simulink model "the_museum"  (R2016b)
settings: Solver=VariableStepAuto  StartTime=0.0  StopTime=10.0  RelTol=1e-3
undefined symbols (not defined in the file or in its folder): Lb, Lf, Lu, RobotStruct
libraries: simulink x1
settings Model: Creator=niekbeckers  LastModifiedBy=Labuser

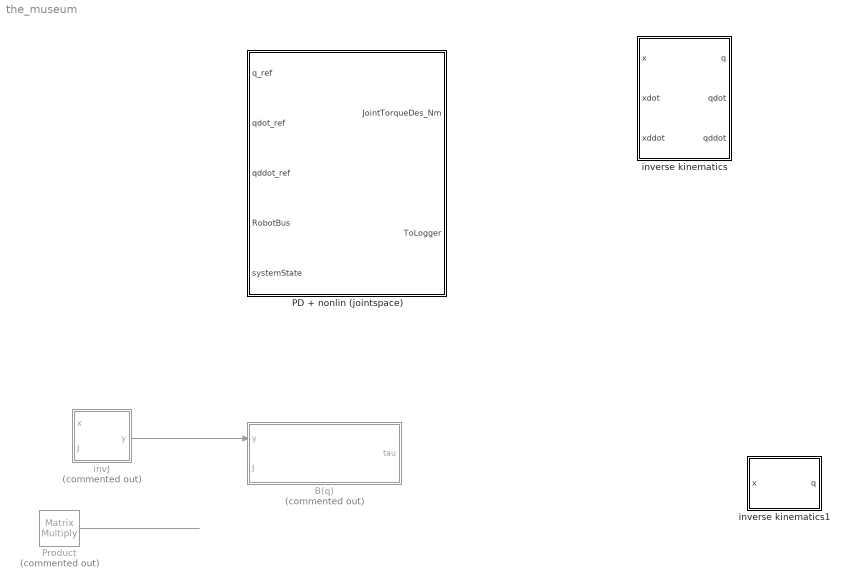
== system the_museum ==
  B(q) : MATLAB Function  Commented=on  TreatAsAtomicUnit=on
  PD + nonlin (jointspace) : Subsystem
  Product : Product  Commented=on  Multiplication=Matrix(*)
  invJ : MATLAB Function  Commented=on  TreatAsAtomicUnit=on
  inverse kinematics : MATLAB Function  TreatAsAtomicUnit=on
  inverse kinematics1 : MATLAB Function  TreatAsAtomicUnit=on
  wires:
  invJ/1(y) -> B(q)/1(y)
  Product/1 -> ?

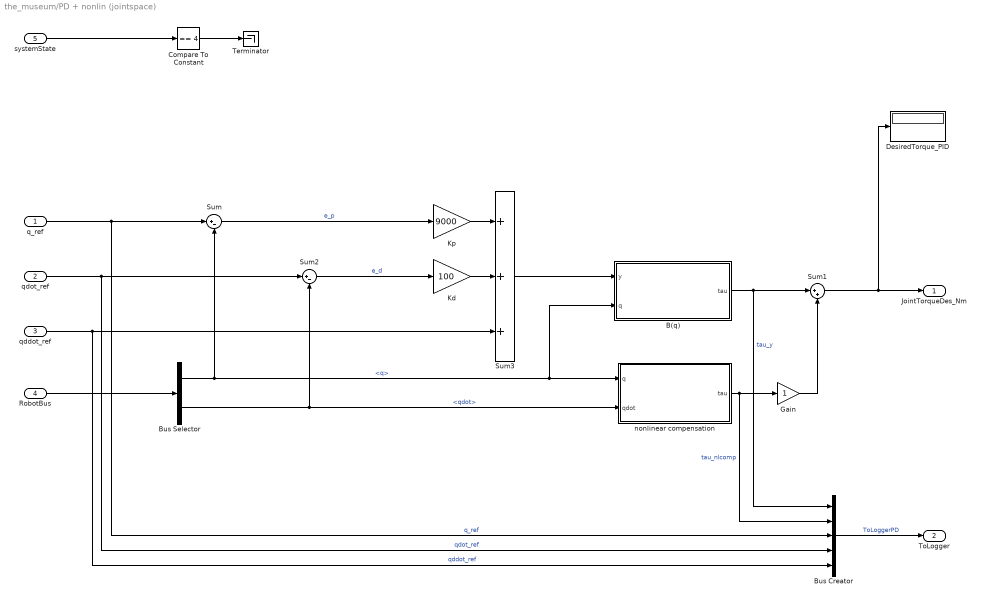
== system the_museum/PD + nonlin (jointspace) ==
  q_ref : Inport
  qdot_ref : Inport  Port=2
  qddot_ref : Inport  Port=3
  RobotBus : Inport  Port=4
  systemState : Inport  Port=5
  B(q) : MATLAB Function  TreatAsAtomicUnit=on
  Bus Creator : BusCreator  Inputs=5
  Bus Selector : BusSelector  OutputSignals=qJointSpace.q,qJointSpace.qdot
  Compare To Constant : simulink/Logic and Bit Operations/Compare To Constant  relop===  const=4  OutDataTypeStr=boolean
  DesiredTorque_PID : Display
  Gain : Gain
  Kd : Gain  Gain=100
  Kp : Gain  Gain=9000
  Sum : Sum  Inputs=|+-
  Sum1 : Sum  Inputs=|++
  Sum2 : Sum  Inputs=|+-
  Sum3 : Sum  Inputs=+++
  Terminator : Terminator
  nonlinear compensation : MATLAB Function  TreatAsAtomicUnit=on
  JointTorqueDes_Nm : Outport
  ToLogger : Outport  Port=2
  wires:
  nonlinear compensation/1(tau) -> Gain/1, Bus Creator/2  "tau_nlcomp"
  B(q)/1(tau) -> Sum1/1, Bus Creator/1  "tau_y"
  Sum3/1 -> B(q)/1(y)
  Kd/1 -> Sum3/2
  Kp/1 -> Sum3/1
  Bus Selector/2 -> nonlinear compensation/2(qdot), Sum2/2  "<qdot>"
  Bus Selector/1 -> Sum/2, nonlinear compensation/1(q), B(q)/2(q)  "<q>"
  q_ref/1 -> Bus Creator/3, Sum/1  "q_ref"
  Sum/1 -> Kp/1  "e_p"
  qdot_ref/1 -> Bus Creator/4, Sum2/1  "qdot_ref"
  Sum2/1 -> Kd/1  "e_d"
  Sum1/1 -> JointTorqueDes_Nm/1, DesiredTorque_PID/1
  RobotBus/1 -> Bus Selector/1
  qddot_ref/1 -> Bus Creator/5, Sum3/3  "qddot_ref"
  systemState/1 -> Compare To Constant/1
  Compare To Constant/1 -> Terminator/1
  Bus Creator/1 -> ToLogger/1  "ToLoggerPD"
  Gain/1 -> Sum1/2

== matlab function the_museum/B(q) ==
  data: y input; J input; tau output; RobotStruct parameter
function tau = Bq(y, J, RobotStruct)
% mass matrix
phat = RobotStruct.DynModParams;

% select parameters
I1 = phat(1);
I2 = phat(2);
me = phat(3);

% jacobian
% J = func_eq_Je(q(1),q(2),Lf,Lu,Lb);

% calculate joint space mass matrix;
I = diag([I1 I2]) + me*(J'*J);

% torque
tau = I*y;

== matlab function the_museum/inverse kinematics ==
  data: x input; xdot input; xddot input; q output size=[2 1]; Lf parameter; Lu parameter; Lb parameter; qdot output; qddot output
function [q,qdot,qddot] = IK(x,xdot,xddot,Lf,Lu,Lb)
%#codegen

% inverse dynamics
q = func_eq_IK(x(1),x(2),Lf,Lu,Lb);

% jacobians
Je = func_eq_Je(q(1),q(2),Lf,Lu,Lb);

% calculate qdot
qdot = pinv(Je)*xdot;

% calculate qddot
Jedot = func_eq_Jedot(q(1),q(2),qdot(1),qdot(2),Lf,Lu,Lb);
qddot = pinv(Je)*(xddot-Jedot*qdot);

== matlab function the_museum/invJ ==
  data: x input; J input; y output
function y = invJ(x,J)

y = pinv(J)*x;

== matlab function the_museum/inverse kinematics1 ==
  data: x input; q output size=[2 1]; Lf parameter; Lu parameter; Lb parameter
function q  = IK(x,Lf,Lu,Lb)
%#codegen

% inverse dynamics
q = func_eq_IK(x(1),x(2),Lf,Lu,Lb);

== matlab function the_museum/PD + nonlin (jointspace)/B(q) ==
  data: y input; q input; tau output; RobotStruct parameter; Lf parameter; Lu parameter; Lb parameter
function tau = Bq(y, q, RobotStruct, Lf, Lu, Lb)
% mass matrix
phat = RobotStruct.DynModParams;

% select parameters
I1 = phat(1);
I2 = phat(2);
me = phat(3);

% jacobian
J = func_eq_Je(q(1),q(2),Lf,Lu,Lb);

% calculate joint space mass matrix;
I = diag([I1 I2]) + me*(J'*J);

% torque
tau = I*y;

== matlab function the_museum/PD + nonlin (jointspace)/nonlinear compensation ==
  data: q input; qdot input; tau output; RobotStruct parameter; Lf parameter; Lu parameter; Lb parameter
function tau = n(q, qdot, RobotStruct, Lf, Lu, Lb)
% mass matrix
phat = RobotStruct.DynModParams;

% select parameters
me = phat(3);
Fs1 = phat(4);
Fv1 = phat(5);
Fs2 = phat(6);
Fv2 = phat(7);

% jacobians
J = func_eq_Je(q(1),q(2),Lf,Lu,Lb);
Jdot = func_eq_Jedot(q(1),q(2),qdot(1),qdot(2),Lf,Lu,Lb);

% calculate joint space mass matrix;
p = [me;Fs1;Fv1;Fs2;Fv2];

% psi 
Psi = [(J'*Jdot)*qdot [ssign(qdot(1)) qdot(1); 0 0] [0 0; ssign(qdot(2)) qdot(2)]];

% torque
tau = Psi*p;

function x = ssign(u,b)
%% x = ssign(u,b)
% soft sign
if nargin < 2
    b = 2;
end

x = 2./(1+exp(-b*u))-1;
